simulink model "D53_LKAS_JLU_20200909_1612"  (R2018b)
settings: Solver=ode3  StartTime=0.0  StopTime=10.0  FixedStep=0.01  RelTol=1e-3  EnableMultiTasking=on
model workspace (MAT data in the model file):
  MCOS : class17 (value not decoded)
  MCOS : class17 (value not decoded)
  MCOS : class17 (value not decoded)
  MCOS : class17 (value not decoded)
  MCOS : class17 (value not decoded)
  MCOS : class17 (value not decoded)
  MCOS : class17 (value not decoded)
  MCOS : class17 (value not decoded)
  MCOS : class17 (value not decoded)
  MCOS : class17 (value not decoded)
  MCOS : class17 (value not decoded)
  MCOS : class17 (value not decoded)
  MCOS : class17 (value not decoded)
  MCOS : class17 (value not decoded)
  MCOS : class17 (value not decoded)
  MCOS : class17 (value not decoded)
  MCOS : class17 (value not decoded)
  MCOS : class17 (value not decoded)
  MCOS : class17 (value not decoded)
  MCOS : class17 (value not decoded)
  MCOS : class17 (value not decoded)
  MCOS : class17 (value not decoded)
  MCOS : class17 (value not decoded)
  MCOS : class17 (value not decoded)
  MCOS : class17 (value not decoded)
  MCOS : class17 (value not decoded)
  MCOS : class17 (value not decoded)
  MCOS : class17 (value not decoded)
  MCOS : class17 (value not decoded)
  MCOS : class17 (value not decoded)
  MCOS : class17 (value not decoded)
  MCOS : class17 (value not decoded)
  MCOS : class17 (value not decoded)
  MCOS : class17 (value not decoded)
  MCOS : class17 (value not decoded)
  MCOS : class17 (value not decoded)
  MCOS : class17 (value not decoded)
  MCOS : class17 (value not decoded)
  MCOS : class17 (value not decoded)
  MCOS : class17 (value not decoded)
  MCOS : class17 (value not decoded)
  MCOS : class17 (value not decoded)
  MCOS : class17 (value not decoded)
  MCOS : class17 (value not decoded)
  MCOS : class17 (value not decoded)
  MCOS : class17 (value not decoded)
  MCOS : class17 (value not decoded)
  MCOS : class17 (value not decoded)
  MCOS : class17 (value not decoded)
  MCOS : class17 (value not decoded)
  MCOS : class17 (value not decoded)
  MCOS : class17 (value not decoded)
  MCOS : class17 (value not decoded)
  MCOS : class17 (value not decoded)
  MCOS : class17 (value not decoded)
  MCOS : class17 (value not decoded)
  MCOS : class17 (value not decoded)
  MCOS : class17 (value not decoded)
  MCOS : class17 (value not decoded)
  MCOS : class17 (value not decoded)
  MCOS : class17 (value not decoded)
  MCOS : class17 (value not decoded)
  MCOS : class17 (value not decoded)
  MCOS : class17 (value not decoded)
  MCOS : class17 (value not decoded)
  MCOS : class17 (value not decoded)
  MCOS : class17 (value not decoded)
  MCOS : class17 (value not decoded)
  MCOS : class17 (value not decoded)
  MCOS : class17 (value not decoded)
  MCOS : class17 (value not decoded)
  MCOS : class17 (value not decoded)
  MCOS : class17 (value not decoded)
  MCOS : class17 (value not decoded)
  MCOS : class17 (value not decoded)
  MCOS : class17 (value not decoded)
  MCOS : class17 (value not decoded)
  MCOS : class17 (value not decoded)
  MCOS : class17 (value not decoded)
  MCOS : class17 (value not decoded)
  MCOS : class17 (value not decoded)
  MCOS : class17 (value not decoded)
  MCOS : class17 (value not decoded)
  MCOS : class17 (value not decoded)
  MCOS : class17 (value not decoded)
  MCOS : class17 (value not decoded)
  MCOS : class17 (value not decoded)
  MCOS : class17 (value not decoded)
  MCOS : class17 (value not decoded)
undefined symbols (not defined in the file): LKA_CarWidth, LKA_SampleTime, LKA_StrRatio_C, LKA_Veh2CamL_C, LKA_Veh2CamW_C, LKA_WhlBaseL_C, LL_CompSWA_C, LL_CrvtPrvwT_C, LL_DesDvt_C, LL_DvtComp_C, LL_DvtPrvwT_C, LL_DvtSpdDet_vDvtSpdMin_C, LL_HdAgExT_C, LL_HdAgPrvwT_C, LL_LAccMax_C, LL_LAccRMax_C, LL_LDW_EarliestWarnLine_C, LL_LDW_LatestWarnLine_C, LL_LDWS_SUPPRESS_HEADING, LL_LFClb_TFC_DiffCtlBalance, LL_LFClb_TFC_DiffCtrlMaxSWA, LL_LFClb_TFC_DiffCtrlRatio, LL_LFClb_TFC_facmGainLutGain1_C, LL_LFClb_TFC_facmGainLutGain2_C, LL_LFClb_TFC_facmIntegRatio, LL_LFClb_TFC_facmKlat_C, LL_LFClb_TFC_FfCtlRatio_C, LL_LFClb_TFC_phiIntegCtlMaxSWA_C, LL_LFClb_TFC_tiKlatPrvwT_C, LL_LFClb_TFC_vGainLutVehSpdLwr_C, LL_LFClb_TFC_vGainLutVehSpdUpr_C, LL_LKA_EarliestWarnLine_C, LL_LKA_LatestWarnLine_C, LL_LKAExPrcs_ExitC0Dvt, LL_LKAExPrcs_ExitC0Swt, LL_LKAExPrcs_tiExitTime1, LL_LKAExPrcs_tiExitTime2, LL_LKAExPrcs_tiExitTime3, LL_LKAS_OUT_OF_CONTROL_LAT_VEL, LL_LKAS_OUT_OF_CONTROL_TTLC, LL_LKASWASyn_M0, LL_LKASWASyn_M1, LL_LKASWASyn_M2, LL_LKASWASyn_M3K, LL_LKASWASyn_SWAaddMax, LL_LKASWASyn_T2, LL_LKASWASyn_tiTrqSwaRtTime, LL_LKASWASyn_tiTrqSwaTime, LL_LKASWASyn_TrqMax, LL_LKASWASyn_TrqSwaAddSwt, LL_LKASWASyn_TrqSwaRateDiff, LL_LSpdCompT_C, LL_lStpLngth_C, LL_MAX_DELAY_EPSSTAR_TIME, LL_MAX_DRIVER_TORQUE_DISABLE, LL_MAX_DRIVER_TORQUE_ENABLE, LL_MAX_LANE_WIDTH_DISABLE, LL_MAX_LANE_WIDTH_ENABLE, LL_MAX_LAT_ACC_DISABLE, LL_MAX_LAT_ACC_ENABLE ... (+30)
libraries: simulink x134, canmsglib x50, dspstat3 x3, simulink_extras x1
(part 2 of 17)

== system D53_LKAS_JLU_20200909_1612/CAN Monitor (CANMon)/Input ==
  In1 : Inport
  In2 : Inport  Port=2
  Bus Selector11 : BusSelector  OutputSignals=bsEPSInfo.EPS_LKA_State,bsEPSInfo.EPS_SW_Trq,bsSWAInfo.SW_Angle,bsSWAInfo.SW_Angle_Speed
  Bus Selector12 : BusSelector  OutputSignals=bsMP5Info.LKA_Main_Switch,bsMP5Info.LKA_Mode,bsPTState.TCU_ActualGear,bsLaneInfo.bsOriL0Info.O_L0_Q,bsLaneInfo.bsOriR0Info.O_R0_Q
  Bus Selector2 : BusSelector  OutputSignals=bsLaneInfo.bsOriL0Info.O_L0_C0,bsLaneInfo.bsOriL0Info.O_L0_C1,bsLaneInfo.bsOriL0Info.O_L0_C2,bsLaneInfo.bsOriL0Info.O_L0_TLC
  Bus Selector7 : BusSelector  OutputSignals=bsLaneInfo.bsOriR0Info.O_R0_C0,bsLaneInfo.bsOriR0Info.O_R0_C1,bsLaneInfo.bsOriR0Info.O_R0_C2,bsLaneInfo.bsOriR0Info.O_R0_TLC
  Bus Selector8 : BusSelector  OutputSignals=bsVehMovInfo.ESC_LatAcc,bsVehMovInfo.ESC_LonAcc,bsVehMovInfo.ESC_VehSpd,bsVehMovInfo.ESC_YawRate
  CAN Pack{16..19} (4 alike) : canmsglib/CAN Pack  CANdbFile=C:\Users\Administrator\Desktop\data_collect.dbc  MsgList=(none)  MsgName=c1deg  MsgIDType=Standard (11-bit identifier)  MsgIdentifier=2022  MsgLength=8  SignalInfo=EPSRx_trgSWTrq$8$16$2$2$1$0$0.01$0$-320$320$#EPSRx_stEPSCtlState$24$16$2$1$1$0$0.01$0$-320$320$#L0Range$40$16$2$1$1$0$1.000000e-002$0$-320$320$#R0Range$56$16$2$1$1$0$1.000000e-002$0$-320$320$#  NSignals=4  StartBits=str2num('[int32(8);int32(24);int32(40);int32(56)]')  SignalSizes=str2num('[int32(16);int32(16);int32(16);int32(16)]')  ByteOrders=str2num('[int32(2);int32(2);int32(2);int32(2)]')  DataTypes=str2num('[int32(2);int32(1);int32(1);int32(1)]')  MultiplexTypes=str2num('[int32(1);int32(1);int32(1);int32(1)]')  MultiplexValues=str2num('[double(0);double(0);double(0);double(0)]')  Factors=str2num('[double(0.01);double(0.01);double(1.000000e-002);double(1.000000e-002)]')  Offsets=str2num('[double(0);double(0);double(0);double(0)]')  Minimums=str2num('[double(-320);double(-320);double(-320);double(-320)]')  Maximums=str2num('[double(320);double(320);double(320);double(320)]')  Remote=off  ApplyMinMax=off  BusOutput=off
      settings: SourceProductName=Simulink Real-Time  SourceProductBaseCode=XP  DataFormat=manually specified signals
  CAN Pack20 : canmsglib/CAN Pack  CANdbFile=F:\LD\1_simulink\GateWay_20180716\dbc\camera_data_in.dbc  MsgList=(none)  MsgName=Video_Lane_Left_A  MsgIDType=Standard (11-bit identifier)  MsgIdentifier=1530  MsgLength=8  SignalInfo=C0$44$12$2$1$1$0$0.000001$0$-3$3$#C1$50$10$2$1$1$0$0.000001$0$-1$1$#C2$24$16$2$1$1$0$0.000001$0$-1$1$#C3$8$16$2$1$1$0$0.000001$0$-1$1$#Line_Type$59$3$2$2$1$0$1$0$0$7$#Message_Counter$48$2$2$2$1$0$1$0$0$3$#Quality$62$2$2$2$1$0$1$0$0$3$#  NSignals=7  StartBits=str2num('[int32(44);int32(50);int32(24);int32(8);int32(59);int32(48);int32(62)]')  SignalSizes=str2num('[int32(12);int32(10);int32(16);int32(16);int32(3);int32(2);int32(2)]')  ByteOrders=str2num('[int32(2);int32(2);int32(2);int32(2);int32(2);int32(2);int32(2)]')  DataTypes=str2num('[int32(1);int32(1);int32(1);int32(1);int32(2);int32(2);int32(2)]')  MultiplexTypes=str2num('[int32(1);int32(1);int32(1);int32(1);int32(1);int32(1);int32(1)]')  MultiplexValues=str2num('[double(0);double(0);double(0);double(0);double(0);double(0);double(0)]')  Factors=str2num('[double(0.000001);double(0.000001);double(0.000001);double(0.000001);double(1);double(1);double(1)]')  Offsets=str2num('[double(0);double(0);double(0);double(0);double(0);double(0);double(0)]')  Minimums=str2num('[double(-3);double(-1);double(-1);double(-1);double(0);double(0);double(0)]')  Maximums=str2num('[double(3);double(1);double(1);double(1);double(7);double(3);double(3)]')  Remote=off  ApplyMinMax=off  BusOutput=off
      settings: SourceProductName=Simulink Real-Time  SourceProductBaseCode=XP  DataFormat=manually specified signals
  CAN Send16 : S-Function  FunctionName=CAN_Send_P  Parameters=uint8(CAN_Port-1),uint8(CAN_Priority-1),uint8(S_overflow_flag),uint8(S_timestamp),double(sampletime)  SFunctionDeploymentMode=off  EnableBusSupport=off  mask{CAN_Port=CAN_0, CAN_Priority=3, S_overflow_flag=off, S_timestamp=off, sampletime=0.01}
      mask prompts: CAN_Port "CAN Port:"; CAN_Priority "Priority:"; S_overflow_flag "Send overflow flag"; S_timestamp "Send time stamp"
      mask init:
      | maskdisplay = cansendicon(CAN_Port,CAN_Priority,S_overflow_flag,S_timestamp);
      | set_param(gcb, 'MaskDisplay', maskdisplay);
      mask TypeOptions CAN_Port: CAN_0 | CAN_1 | CAN_2 | CAN_3
      mask TypeOptions CAN_Priority: 0 | 1 | 2 | 3 | 4 | 5 | 6 | 7
      mask Display: color('blue');text(0.98,0.9,'MPC5675K','horizontalAlignment','right');color('black');text(0.5,0.6,'FlexCAN_0 Send','horizontalAlignment','center');text(0.5,0.35,'Priority:3','horizontalAlignment','center');port_label('input',1,'CAN_Msg');
  CAN Send17 : S-Function  FunctionName=CAN_Send_P  Parameters=uint8(CAN_Port-1),uint8(CAN_Priority-1),uint8(S_overflow_flag),uint8(S_timestamp),double(sampletime)  SFunctionDeploymentMode=off  EnableBusSupport=off  mask{CAN_Port=CAN_0, CAN_Priority=3, S_overflow_flag=off, S_timestamp=off, sampletime=0.01}
      mask prompts: CAN_Port "CAN Port:"; CAN_Priority "Priority:"; S_overflow_flag "Send overflow flag"; S_timestamp "Send time stamp"
      mask init:
      | maskdisplay = cansendicon(CAN_Port,CAN_Priority,S_overflow_flag,S_timestamp);
      | set_param(gcb, 'MaskDisplay', maskdisplay);
      mask TypeOptions CAN_Port: CAN_0 | CAN_1 | CAN_2 | CAN_3
      mask TypeOptions CAN_Priority: 0 | 1 | 2 | 3 | 4 | 5 | 6 | 7
      mask Display: color('blue');text(0.98,0.9,'MPC5675K','horizontalAlignment','right');color('black');text(0.5,0.6,'FlexCAN_0 Send','horizontalAlignment','center');text(0.5,0.35,'Priority:3','horizontalAlignment','center');port_label('input',1,'CAN_Msg');
  CAN Send18 : S-Function  FunctionName=CAN_Send_P  Parameters=uint8(CAN_Port-1),uint8(CAN_Priority-1),uint8(S_overflow_flag),uint8(S_timestamp),double(sampletime)  SFunctionDeploymentMode=off  EnableBusSupport=off  mask{CAN_Port=CAN_0, CAN_Priority=3, S_overflow_flag=off, S_timestamp=off, sampletime=0.01}
      mask prompts: CAN_Port "CAN Port:"; CAN_Priority "Priority:"; S_overflow_flag "Send overflow flag"; S_timestamp "Send time stamp"
      mask init:
      | maskdisplay = cansendicon(CAN_Port,CAN_Priority,S_overflow_flag,S_timestamp);
      | set_param(gcb, 'MaskDisplay', maskdisplay);
      mask TypeOptions CAN_Port: CAN_0 | CAN_1 | CAN_2 | CAN_3
      mask TypeOptions CAN_Priority: 0 | 1 | 2 | 3 | 4 | 5 | 6 | 7
      mask Display: color('blue');text(0.98,0.9,'MPC5675K','horizontalAlignment','right');color('black');text(0.5,0.6,'FlexCAN_0 Send','horizontalAlignment','center');text(0.5,0.35,'Priority:3','horizontalAlignment','center');port_label('input',1,'CAN_Msg');
  CAN Send19 : S-Function  FunctionName=CAN_Send_P  Parameters=uint8(CAN_Port-1),uint8(CAN_Priority-1),uint8(S_overflow_flag),uint8(S_timestamp),double(sampletime)  SFunctionDeploymentMode=off  EnableBusSupport=off  mask{CAN_Port=CAN_0, CAN_Priority=3, S_overflow_flag=off, S_timestamp=off, sampletime=0.01}
      mask prompts: CAN_Port "CAN Port:"; CAN_Priority "Priority:"; S_overflow_flag "Send overflow flag"; S_timestamp "Send time stamp"
      mask init:
      | maskdisplay = cansendicon(CAN_Port,CAN_Priority,S_overflow_flag,S_timestamp);
      | set_param(gcb, 'MaskDisplay', maskdisplay);
      mask TypeOptions CAN_Port: CAN_0 | CAN_1 | CAN_2 | CAN_3
      mask TypeOptions CAN_Priority: 0 | 1 | 2 | 3 | 4 | 5 | 6 | 7
      mask Display: color('blue');text(0.98,0.9,'MPC5675K','horizontalAlignment','right');color('black');text(0.5,0.6,'FlexCAN_0 Send','horizontalAlignment','center');text(0.5,0.35,'Priority:3','horizontalAlignment','center');port_label('input',1,'CAN_Msg');
  CAN Send20 : S-Function  FunctionName=CAN_Send_P  Parameters=uint8(CAN_Port-1),uint8(CAN_Priority-1),uint8(S_overflow_flag),uint8(S_timestamp),double(sampletime)  SFunctionDeploymentMode=off  EnableBusSupport=off  mask{CAN_Port=CAN_0, CAN_Priority=3, S_overflow_flag=off, S_timestamp=off, sampletime=0.01}
      mask prompts: CAN_Port "CAN Port:"; CAN_Priority "Priority:"; S_overflow_flag "Send overflow flag"; S_timestamp "Send time stamp"
      mask init:
      | maskdisplay = cansendicon(CAN_Port,CAN_Priority,S_overflow_flag,S_timestamp);
      | set_param(gcb, 'MaskDisplay', maskdisplay);
      mask TypeOptions CAN_Port: CAN_0 | CAN_1 | CAN_2 | CAN_3
      mask TypeOptions CAN_Priority: 0 | 1 | 2 | 3 | 4 | 5 | 6 | 7
      mask Display: color('blue');text(0.98,0.9,'MPC5675K','horizontalAlignment','right');color('black');text(0.5,0.6,'FlexCAN_0 Send','horizontalAlignment','center');text(0.5,0.35,'Priority:3','horizontalAlignment','center');port_label('input',1,'CAN_Msg');
  Data Type Conversion{54..69} (16 alike) : DataTypeConversion  OutDataTypeStr=single
  Data Type Conversion{70..74} (5 alike) : DataTypeConversion  OutDataTypeStr=uint8
  wires:
  Data Type Conversion59/1 -> CAN Pack17/2
  Data Type Conversion60/1 -> CAN Pack17/3
  Bus Selector2/1 -> Data Type Conversion54/1  "<O_L0_C0>"
  Bus Selector12/1 -> Data Type Conversion70/1  "<LKA_Main_Switch>"
  CAN Pack18/1 -> CAN Send18/1
  Data Type Conversion66/1 -> CAN Pack19/1
  Data Type Conversion71/1 -> CAN Pack20/2
  [bsInInfo] -> Bus Selector7/1
  Data Type Conversion72/1 -> CAN Pack20/3
  Bus Selector12/4 -> Data Type Conversion73/1  "<O_L0_Q>"
  [bsInInfo] -> Bus Selector8/1
  Bus Selector2/2 -> Data Type Conversion55/1  "<O_L0_C1>"
  Data Type Conversion55/1 -> CAN Pack16/2
  Data Type Conversion57/1 -> CAN Pack16/4
  Bus Selector11/2 -> Data Type Conversion67/1  "<EPS_SW_Trq>"
  Bus Selector12/2 -> Data Type Conversion71/1  "<LKA_Mode>"
  Data Type Conversion61/1 -> CAN Pack17/4
  Bus Selector12/3 -> Data Type Conversion72/1  "<TCU_ActualGear>"
  In1/1 -> CAN Pack20/6
  Data Type Conversion64/1 -> CAN Pack18/3
  CAN Pack20/1 -> CAN Send20/1
  Bus Selector8/3 -> Data Type Conversion64/1  "<ESC_VehSpd>"
  Bus Selector8/4 -> Data Type Conversion65/1  "<ESC_YawRate>"
  Bus Selector7/1 -> Data Type Conversion58/1  "<O_R0_C0>"
  Bus Selector8/2 -> Data Type Conversion63/1  "<ESC_LonAcc>"
  In2/1 -> CAN Pack20/7
  Bus Selector7/2 -> Data Type Conversion59/1  "<O_R0_C1>"
  Bus Selector7/4 -> Data Type Conversion61/1  "<O_R0_TLC>"
  Bus Selector11/3 -> Data Type Conversion68/1  "<SW_Angle>"
  Bus Selector11/4 -> Data Type Conversion69/1  "<SW_Angle_Speed>"
  CAN Pack16/1 -> CAN Send16/1
  Data Type Conversion56/1 -> CAN Pack16/3
  Data Type Conversion70/1 -> CAN Pack20/1
  Bus Selector11/1 -> Data Type Conversion66/1  "<EPS_LKA_State>"
  Bus Selector2/3 -> Data Type Conversion56/1  "<O_L0_C2>"
  Bus Selector12/5 -> Data Type Conversion74/1  "<O_R0_Q>"
  Bus Selector8/1 -> Data Type Conversion62/1  "<ESC_LatAcc>"
  CAN Pack17/1 -> CAN Send17/1
  [bsInInfo] -> Bus Selector11/1
  Data Type Conversion58/1 -> CAN Pack17/1
  [bsInInfo] -> Bus Selector2/1
  Bus Selector7/3 -> Data Type Conversion60/1  "<O_R0_C2>"
  Bus Selector2/4 -> Data Type Conversion57/1  "<O_L0_TLC>"
  Data Type Conversion68/1 -> CAN Pack19/3
  Data Type Conversion54/1 -> CAN Pack16/1
  Data Type Conversion74/1 -> CAN Pack20/5
  CAN Pack19/1 -> CAN Send19/1
  [bsInInfo] -> Bus Selector12/1
  Data Type Conversion65/1 -> CAN Pack18/4
  Data Type Conversion63/1 -> CAN Pack18/2
  Data Type Conversion73/1 -> CAN Pack20/4
  Data Type Conversion67/1 -> CAN Pack19/2
  Data Type Conversion69/1 -> CAN Pack19/4
  Data Type Conversion62/1 -> CAN Pack18/1

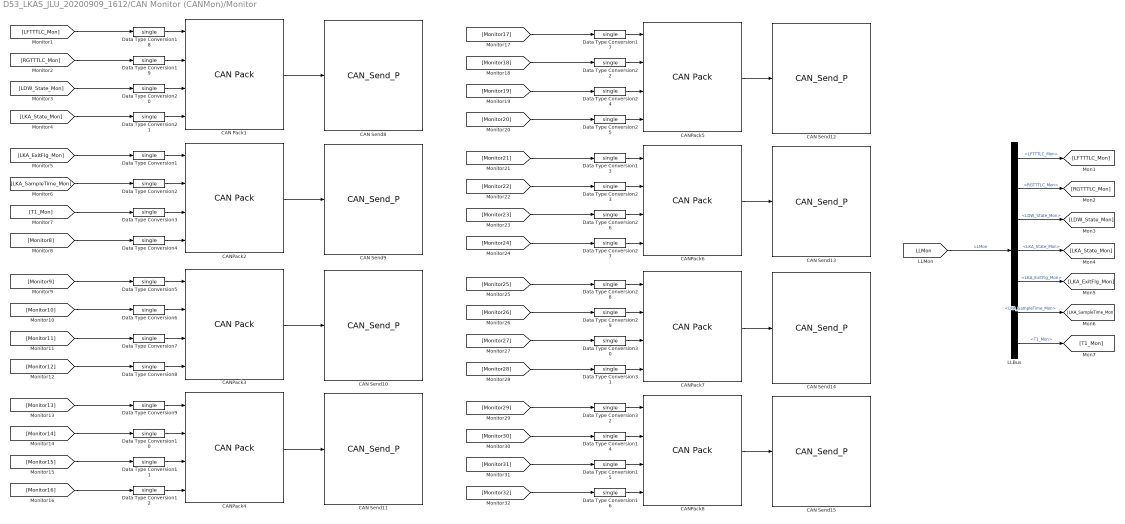
== system D53_LKAS_JLU_20200909_1612/CAN Monitor (CANMon)/Monitor ==
  CAN Pack1 : canmsglib/CAN Pack  CANdbFile=D:\LKAS\Documents\LKAS-Monitor.dbc  MsgList=Mon_1  MsgName=Mon_1  MsgIDType=Standard (11-bit identifier)  MsgIdentifier=1536  MsgLength=8  SignalInfo=Signal_1$8$16$2$1$1$0$1.000000e-02$0$-3.276800e+02$3.276700e+02$#Signal_2$24$16$2$1$1$0$1.000000e-02$0$-3.276800e+02$3.276700e+02$#Signal_3$40$16$2$1$1$0$1.000000e-02$0$-3.276800e+02$3.276700e+02$#Signal_4$56$16$2$1$1$0$1.000000e-02$0$-3.276800e+02$3.276700e+02$#  NSignals=4  StartBits=str2num('[int32(8);int32(24);int32(40);int32(56)]')  SignalSizes=str2num('[int32(16);int32(16);int32(16);int32(16)]')  ByteOrders=str2num('[int32(2);int32(2);int32(2);int32(2)]')  DataTypes=str2num('[int32(1);int32(1);int32(1);int32(1)]')  MultiplexTypes=str2num('[int32(1);int32(1);int32(1);int32(1)]')  MultiplexValues=str2num('[double(0);double(0);double(0);double(0)]')  Factors=str2num('[double(1.000000e-02);double(1.000000e-02);double(1.000000e-02);double(1.000000e-02)]')  Offsets=str2num('[double(0);double(0);double(0);double(0)]')  Minimums=str2num('[double(-3.276800e+02);double(-3.276800e+02);double(-3.276800e+02);double(-3.276800e+02)]')  Maximums=str2num('[double(3.276700e+02);double(3.276700e+02);double(3.276700e+02);double(3.276700e+02)]')  Remote=off  ApplyMinMax=off  BusOutput=off
      settings: SourceProductName=Simulink Real-Time  SourceProductBaseCode=XP  DataFormat=CANdb specified signals
  CAN Send10 : S-Function  FunctionName=CAN_Send_P  Parameters=uint8(CAN_Port-1),uint8(CAN_Priority-1),uint8(S_overflow_flag),uint8(S_timestamp),double(sampletime)  SFunctionDeploymentMode=off  EnableBusSupport=off  mask{CAN_Port=CAN_0, CAN_Priority=3, S_overflow_flag=off, S_timestamp=off, sampletime=0.01}
      mask prompts: CAN_Port "CAN Port:"; CAN_Priority "Priority:"; S_overflow_flag "Send overflow flag"; S_timestamp "Send time stamp"
      mask init:
      | maskdisplay = cansendicon(CAN_Port,CAN_Priority,S_overflow_flag,S_timestamp);
      | set_param(gcb, 'MaskDisplay', maskdisplay);
      mask TypeOptions CAN_Port: CAN_0 | CAN_1 | CAN_2 | CAN_3
      mask TypeOptions CAN_Priority: 0 | 1 | 2 | 3 | 4 | 5 | 6 | 7
      mask Display: color('blue');text(0.98,0.9,'MPC5675K','horizontalAlignment','right');color('black');text(0.5,0.6,'FlexCAN_0 Send','horizontalAlignment','center');text(0.5,0.35,'Priority:3','horizontalAlignment','center');port_label('input',1,'CAN_Msg');
  CAN Send11 : S-Function  FunctionName=CAN_Send_P  Parameters=uint8(CAN_Port-1),uint8(CAN_Priority-1),uint8(S_overflow_flag),uint8(S_timestamp),double(sampletime)  SFunctionDeploymentMode=off  EnableBusSupport=off  mask{CAN_Port=CAN_0, CAN_Priority=3, S_overflow_flag=off, S_timestamp=off, sampletime=0.01}
      mask prompts: CAN_Port "CAN Port:"; CAN_Priority "Priority:"; S_overflow_flag "Send overflow flag"; S_timestamp "Send time stamp"
      mask init:
      | maskdisplay = cansendicon(CAN_Port,CAN_Priority,S_overflow_flag,S_timestamp);
      | set_param(gcb, 'MaskDisplay', maskdisplay);
      mask TypeOptions CAN_Port: CAN_0 | CAN_1 | CAN_2 | CAN_3
      mask TypeOptions CAN_Priority: 0 | 1 | 2 | 3 | 4 | 5 | 6 | 7
      mask Display: color('blue');text(0.98,0.9,'MPC5675K','horizontalAlignment','right');color('black');text(0.5,0.6,'FlexCAN_0 Send','horizontalAlignment','center');text(0.5,0.35,'Priority:3','horizontalAlignment','center');port_label('input',1,'CAN_Msg');
  CAN Send12 : S-Function  FunctionName=CAN_Send_P  Parameters=uint8(CAN_Port-1),uint8(CAN_Priority-1),uint8(S_overflow_flag),uint8(S_timestamp),double(sampletime)  SFunctionDeploymentMode=off  EnableBusSupport=off  mask{CAN_Port=CAN_0, CAN_Priority=3, S_overflow_flag=off, S_timestamp=off, sampletime=0.01}
      mask prompts: CAN_Port "CAN Port:"; CAN_Priority "Priority:"; S_overflow_flag "Send overflow flag"; S_timestamp "Send time stamp"
      mask init:
      | maskdisplay = cansendicon(CAN_Port,CAN_Priority,S_overflow_flag,S_timestamp);
      | set_param(gcb, 'MaskDisplay', maskdisplay);
      mask TypeOptions CAN_Port: CAN_0 | CAN_1 | CAN_2 | CAN_3
      mask TypeOptions CAN_Priority: 0 | 1 | 2 | 3 | 4 | 5 | 6 | 7
      mask Display: color('blue');text(0.98,0.9,'MPC5675K','horizontalAlignment','right');color('black');text(0.5,0.6,'FlexCAN_0 Send','horizontalAlignment','center');text(0.5,0.35,'Priority:3','horizontalAlignment','center');port_label('input',1,'CAN_Msg');
  CAN Send13 : S-Function  FunctionName=CAN_Send_P  Parameters=uint8(CAN_Port-1),uint8(CAN_Priority-1),uint8(S_overflow_flag),uint8(S_timestamp),double(sampletime)  SFunctionDeploymentMode=off  EnableBusSupport=off  mask{CAN_Port=CAN_0, CAN_Priority=3, S_overflow_flag=off, S_timestamp=off, sampletime=0.01}
      mask prompts: CAN_Port "CAN Port:"; CAN_Priority "Priority:"; S_overflow_flag "Send overflow flag"; S_timestamp "Send time stamp"
      mask init:
      | maskdisplay = cansendicon(CAN_Port,CAN_Priority,S_overflow_flag,S_timestamp);
      | set_param(gcb, 'MaskDisplay', maskdisplay);
      mask TypeOptions CAN_Port: CAN_0 | CAN_1 | CAN_2 | CAN_3
      mask TypeOptions CAN_Priority: 0 | 1 | 2 | 3 | 4 | 5 | 6 | 7
      mask Display: color('blue');text(0.98,0.9,'MPC5675K','horizontalAlignment','right');color('black');text(0.5,0.6,'FlexCAN_0 Send','horizontalAlignment','center');text(0.5,0.35,'Priority:3','horizontalAlignment','center');port_label('input',1,'CAN_Msg');
  CAN Send14 : S-Function  FunctionName=CAN_Send_P  Parameters=uint8(CAN_Port-1),uint8(CAN_Priority-1),uint8(S_overflow_flag),uint8(S_timestamp),double(sampletime)  SFunctionDeploymentMode=off  EnableBusSupport=off  mask{CAN_Port=CAN_0, CAN_Priority=3, S_overflow_flag=off, S_timestamp=off, sampletime=0.01}
      mask prompts: CAN_Port "CAN Port:"; CAN_Priority "Priority:"; S_overflow_flag "Send overflow flag"; S_timestamp "Send time stamp"
      mask init:
      | maskdisplay = cansendicon(CAN_Port,CAN_Priority,S_overflow_flag,S_timestamp);
      | set_param(gcb, 'MaskDisplay', maskdisplay);
      mask TypeOptions CAN_Port: CAN_0 | CAN_1 | CAN_2 | CAN_3
      mask TypeOptions CAN_Priority: 0 | 1 | 2 | 3 | 4 | 5 | 6 | 7
      mask Display: color('blue');text(0.98,0.9,'MPC5675K','horizontalAlignment','right');color('black');text(0.5,0.6,'FlexCAN_0 Send','horizontalAlignment','center');text(0.5,0.35,'Priority:3','horizontalAlignment','center');port_label('input',1,'CAN_Msg');
  CAN Send15 : S-Function  FunctionName=CAN_Send_P  Parameters=uint8(CAN_Port-1),uint8(CAN_Priority-1),uint8(S_overflow_flag),uint8(S_timestamp),double(sampletime)  SFunctionDeploymentMode=off  EnableBusSupport=off  mask{CAN_Port=CAN_0, CAN_Priority=3, S_overflow_flag=off, S_timestamp=off, sampletime=0.01}
      mask prompts: CAN_Port "CAN Port:"; CAN_Priority "Priority:"; S_overflow_flag "Send overflow flag"; S_timestamp "Send time stamp"
      mask init:
      | maskdisplay = cansendicon(CAN_Port,CAN_Priority,S_overflow_flag,S_timestamp);
      | set_param(gcb, 'MaskDisplay', maskdisplay);
      mask TypeOptions CAN_Port: CAN_0 | CAN_1 | CAN_2 | CAN_3
      mask TypeOptions CAN_Priority: 0 | 1 | 2 | 3 | 4 | 5 | 6 | 7
      mask Display: color('blue');text(0.98,0.9,'MPC5675K','horizontalAlignment','right');color('black');text(0.5,0.6,'FlexCAN_0 Send','horizontalAlignment','center');text(0.5,0.35,'Priority:3','horizontalAlignment','center');port_label('input',1,'CAN_Msg');
  CAN Send8 : S-Function  FunctionName=CAN_Send_P  Parameters=uint8(CAN_Port-1),uint8(CAN_Priority-1),uint8(S_overflow_flag),uint8(S_timestamp),double(sampletime)  SFunctionDeploymentMode=off  EnableBusSupport=off  mask{CAN_Port=CAN_0, CAN_Priority=3, S_overflow_flag=off, S_timestamp=off, sampletime=0.01}
      mask prompts: CAN_Port "CAN Port:"; CAN_Priority "Priority:"; S_overflow_flag "Send overflow flag"; S_timestamp "Send time stamp"
      mask init:
      | maskdisplay = cansendicon(CAN_Port,CAN_Priority,S_overflow_flag,S_timestamp);
      | set_param(gcb, 'MaskDisplay', maskdisplay);
      mask TypeOptions CAN_Port: CAN_0 | CAN_1 | CAN_2 | CAN_3
      mask TypeOptions CAN_Priority: 0 | 1 | 2 | 3 | 4 | 5 | 6 | 7
      mask Display: color('blue');text(0.98,0.9,'MPC5675K','horizontalAlignment','right');color('black');text(0.5,0.6,'FlexCAN_0 Send','horizontalAlignment','center');text(0.5,0.35,'Priority:3','horizontalAlignment','center');port_label('input',1,'CAN_Msg');
  CAN Send9 : S-Function  FunctionName=CAN_Send_P  Parameters=uint8(CAN_Port-1),uint8(CAN_Priority-1),uint8(S_overflow_flag),uint8(S_timestamp),double(sampletime)  SFunctionDeploymentMode=off  EnableBusSupport=off  mask{CAN_Port=CAN_0, CAN_Priority=3, S_overflow_flag=off, S_timestamp=off, sampletime=0.01}
      mask prompts: CAN_Port "CAN Port:"; CAN_Priority "Priority:"; S_overflow_flag "Send overflow flag"; S_timestamp "Send time stamp"
      mask init:
      | maskdisplay = cansendicon(CAN_Port,CAN_Priority,S_overflow_flag,S_timestamp);
      | set_param(gcb, 'MaskDisplay', maskdisplay);
      mask TypeOptions CAN_Port: CAN_0 | CAN_1 | CAN_2 | CAN_3
      mask TypeOptions CAN_Priority: 0 | 1 | 2 | 3 | 4 | 5 | 6 | 7
      mask Display: color('blue');text(0.98,0.9,'MPC5675K','horizontalAlignment','right');color('black');text(0.5,0.6,'FlexCAN_0 Send','horizontalAlignment','center');text(0.5,0.35,'Priority:3','horizontalAlignment','center');port_label('input',1,'CAN_Msg');
  CANPack2 : canmsglib/CAN Pack  CANdbFile=D:\LKAS\Documents\LKAS-Monitor.dbc  MsgList=Mon_2  MsgName=Mon_2  MsgIDType=Standard (11-bit identifier)  MsgIdentifier=1552  MsgLength=8  SignalInfo=bsInInfo1$8$16$2$1$1$0$1.000000e-02$0$-3.276800e+02$3.276700e+02$#bsInInfo2$24$16$2$1$1$0$1.000000e-02$0$-3.276800e+02$3.276700e+02$#bsInInfo3$40$16$2$1$1$0$1.000000e-02$0$-3.276800e+02$3.276700e+02$#bsInInfo4$56$16$2$1$1$0$1.000000e-02$0$-3.276800e+02$3.276700e+02$#  NSignals=4  StartBits=str2num('[int32(8);int32(24);int32(40);int32(56)]')  SignalSizes=str2num('[int32(16);int32(16);int32(16);int32(16)]')  ByteOrders=str2num('[int32(2);int32(2);int32(2);int32(2)]')  DataTypes=str2num('[int32(1);int32(1);int32(1);int32(1)]')  MultiplexTypes=str2num('[int32(1);int32(1);int32(1);int32(1)]')  MultiplexValues=str2num('[double(0);double(0);double(0);double(0)]')  Factors=str2num('[double(1.000000e-02);double(1.000000e-02);double(1.000000e-02);double(1.000000e-02)]')  Offsets=str2num('[double(0);double(0);double(0);double(0)]')  Minimums=str2num('[double(-3.276800e+02);double(-3.276800e+02);double(-3.276800e+02);double(-3.276800e+02)]')  Maximums=str2num('[double(3.276700e+02);double(3.276700e+02);double(3.276700e+02);double(3.276700e+02)]')  Remote=off  ApplyMinMax=off  BusOutput=off
      settings: SourceProductName=Simulink Real-Time  SourceProductBaseCode=XP  DataFormat=CANdb specified signals
  CANPack3 : canmsglib/CAN Pack  CANdbFile=D:\LKAS\Documents\LKAS-Monitor.dbc  MsgList=Mon_3  MsgName=Mon_3  MsgIDType=Standard (11-bit identifier)  MsgIdentifier=1568  MsgLength=8  SignalInfo=Signal_10$24$16$2$1$1$0$1.000000e-02$0$-3.276800e+02$3.276700e+02$#Signal_11$40$16$2$1$1$0$1.000000e-02$0$-3.276800e+02$3.276700e+02$#Signal_12$56$16$2$1$1$0$1.000000e-02$0$-3.276800e+02$3.276700e+02$#Signal_9$8$16$2$1$1$0$1.000000e-02$0$-3.276800e+02$3.276700e+02$#  NSignals=4  StartBits=str2num('[int32(24);int32(40);int32(56);int32(8)]')  SignalSizes=str2num('[int32(16);int32(16);int32(16);int32(16)]')  ByteOrders=str2num('[int32(2);int32(2);int32(2);int32(2)]')  DataTypes=str2num('[int32(1);int32(1);int32(1);int32(1)]')  MultiplexTypes=str2num('[int32(1);int32(1);int32(1);int32(1)]')  MultiplexValues=str2num('[double(0);double(0);double(0);double(0)]')  Factors=str2num('[double(1.000000e-02);double(1.000000e-02);double(1.000000e-02);double(1.000000e-02)]')  Offsets=str2num('[double(0);double(0);double(0);double(0)]')  Minimums=str2num('[double(-3.276800e+02);double(-3.276800e+02);double(-3.276800e+02);double(-3.276800e+02)]')  Maximums=str2num('[double(3.276700e+02);double(3.276700e+02);double(3.276700e+02);double(3.276700e+02)]')  Remote=off  ApplyMinMax=off  BusOutput=off
      settings: SourceProductName=Simulink Real-Time  SourceProductBaseCode=XP  DataFormat=CANdb specified signals
  CANPack4 : canmsglib/CAN Pack  CANdbFile=D:\LKAS\Documents\LKAS-Monitor.dbc  MsgList=Mon_4  MsgName=Mon_4  MsgIDType=Standard (11-bit identifier)  MsgIdentifier=1584  MsgLength=8  SignalInfo=Signal_13$8$16$2$1$1$0$1.000000e-02$0$-3.276800e+02$3.276700e+02$#Signal_14$24$16$2$1$1$0$1.000000e-02$0$-3.276800e+02$3.276700e+02$#Signal_15$40$16$2$1$1$0$1.000000e-02$0$-3.276800e+02$3.276700e+02$#Signal_16$56$16$2$1$1$0$1.000000e-02$0$-3.276800e+02$3.276700e+02$#  NSignals=4  StartBits=str2num('[int32(8);int32(24);int32(40);int32(56)]')  SignalSizes=str2num('[int32(16);int32(16);int32(16);int32(16)]')  ByteOrders=str2num('[int32(2);int32(2);int32(2);int32(2)]')  DataTypes=str2num('[int32(1);int32(1);int32(1);int32(1)]')  MultiplexTypes=str2num('[int32(1);int32(1);int32(1);int32(1)]')  MultiplexValues=str2num('[double(0);double(0);double(0);double(0)]')  Factors=str2num('[double(1.000000e-02);double(1.000000e-02);double(1.000000e-02);double(1.000000e-02)]')  Offsets=str2num('[double(0);double(0);double(0);double(0)]')  Minimums=str2num('[double(-3.276800e+02);double(-3.276800e+02);double(-3.276800e+02);double(-3.276800e+02)]')  Maximums=str2num('[double(3.276700e+02);double(3.276700e+02);double(3.276700e+02);double(3.276700e+02)]')  Remote=off  ApplyMinMax=off  BusOutput=off
      settings: SourceProductName=Simulink Real-Time  SourceProductBaseCode=XP  DataFormat=CANdb specified signals
  CANPack5 : canmsglib/CAN Pack  CANdbFile=D:\LKAS\Documents\LKAS-Monitor.dbc  MsgList=Mon_5  MsgName=Mon_5  MsgIDType=Standard (11-bit identifier)  MsgIdentifier=1600  MsgLength=8  SignalInfo=Signal_17$8$16$2$1$1$0$1.000000e-02$0$-3.276800e+02$3.276700e+02$#Signal_18$24$16$2$1$1$0$1.000000e-02$0$-3.276800e+02$3.276700e+02$#Signal_19$40$16$2$1$1$0$1.000000e-02$0$-3.276800e+02$3.276700e+02$#Signal_20$56$16$2$1$1$0$1.000000e-02$0$-3.276800e+02$3.276700e+02$#  NSignals=4  StartBits=str2num('[int32(8);int32(24);int32(40);int32(56)]')  SignalSizes=str2num('[int32(16);int32(16);int32(16);int32(16)]')  ByteOrders=str2num('[int32(2);int32(2);int32(2);int32(2)]')  DataTypes=str2num('[int32(1);int32(1);int32(1);int32(1)]')  MultiplexTypes=str2num('[int32(1);int32(1);int32(1);int32(1)]')  MultiplexValues=str2num('[double(0);double(0);double(0);double(0)]')  Factors=str2num('[double(1.000000e-02);double(1.000000e-02);double(1.000000e-02);double(1.000000e-02)]')  Offsets=str2num('[double(0);double(0);double(0);double(0)]')  Minimums=str2num('[double(-3.276800e+02);double(-3.276800e+02);double(-3.276800e+02);double(-3.276800e+02)]')  Maximums=str2num('[double(3.276700e+02);double(3.276700e+02);double(3.276700e+02);double(3.276700e+02)]')  Remote=off  ApplyMinMax=off  BusOutput=off
      settings: SourceProductName=Simulink Real-Time  SourceProductBaseCode=XP  DataFormat=CANdb specified signals
  CANPack6 : canmsglib/CAN Pack  CANdbFile=D:\LKAS\Documents\LKAS-Monitor.dbc  MsgList=Mon_6  MsgName=Mon_6  MsgIDType=Standard (11-bit identifier)  MsgIdentifier=1616  MsgLength=8  SignalInfo=Signal_21$8$16$2$1$1$0$1.000000e-02$0$-3.276800e+02$3.276700e+02$#Signal_22$24$16$2$1$1$0$1.000000e-02$0$-3.276800e+02$3.276700e+02$#Signal_23$40$16$2$1$1$0$1.000000e-02$0$-3.276800e+02$3.276700e+02$#Signal_24$56$16$2$1$1$0$1.000000e-02$0$-3.276800e+02$3.276700e+02$#  NSignals=4  StartBits=str2num('[int32(8);int32(24);int32(40);int32(56)]')  SignalSizes=str2num('[int32(16);int32(16);int32(16);int32(16)]')  ByteOrders=str2num('[int32(2);int32(2);int32(2);int32(2)]')  DataTypes=str2num('[int32(1);int32(1);int32(1);int32(1)]')  MultiplexTypes=str2num('[int32(1);int32(1);int32(1);int32(1)]')  MultiplexValues=str2num('[double(0);double(0);double(0);double(0)]')  Factors=str2num('[double(1.000000e-02);double(1.000000e-02);double(1.000000e-02);double(1.000000e-02)]')  Offsets=str2num('[double(0);double(0);double(0);double(0)]')  Minimums=str2num('[double(-3.276800e+02);double(-3.276800e+02);double(-3.276800e+02);double(-3.276800e+02)]')  Maximums=str2num('[double(3.276700e+02);double(3.276700e+02);double(3.276700e+02);double(3.276700e+02)]')  Remote=off  ApplyMinMax=off  BusOutput=off
      settings: SourceProductName=Simulink Real-Time  SourceProductBaseCode=XP  DataFormat=CANdb specified signals
  CANPack7 : canmsglib/CAN Pack  CANdbFile=D:\LKAS\Documents\LKAS-Monitor.dbc  MsgList=Mon_7  MsgName=Mon_7  MsgIDType=Standard (11-bit identifier)  MsgIdentifier=1632  MsgLength=8  SignalInfo=Signal_25$8$16$2$1$1$0$1.000000e-02$0$-3.276800e+02$3.276700e+02$#Signal_26$24$16$2$1$1$0$1.000000e-02$0$-3.276800e+02$3.276700e+02$#Signal_27$40$16$2$1$1$0$1.000000e-02$0$-3.276800e+02$3.276700e+02$#Signal_28$56$16$2$1$1$0$1.000000e-02$0$-3.276800e+02$3.276700e+02$#  NSignals=4  StartBits=str2num('[int32(8);int32(24);int32(40);int32(56)]')  SignalSizes=str2num('[int32(16);int32(16);int32(16);int32(16)]')  ByteOrders=str2num('[int32(2);int32(2);int32(2);int32(2)]')  DataTypes=str2num('[int32(1);int32(1);int32(1);int32(1)]')  MultiplexTypes=str2num('[int32(1);int32(1);int32(1);int32(1)]')  MultiplexValues=str2num('[double(0);double(0);double(0);double(0)]')  Factors=str2num('[double(1.000000e-02);double(1.000000e-02);double(1.000000e-02);double(1.000000e-02)]')  Offsets=str2num('[double(0);double(0);double(0);double(0)]')  Minimums=str2num('[double(-3.276800e+02);double(-3.276800e+02);double(-3.276800e+02);double(-3.276800e+02)]')  Maximums=str2num('[double(3.276700e+02);double(3.276700e+02);double(3.276700e+02);double(3.276700e+02)]')  Remote=off  ApplyMinMax=off  BusOutput=off
      settings: SourceProductName=Simulink Real-Time  SourceProductBaseCode=XP  DataFormat=CANdb specified signals
  CANPack8 : canmsglib/CAN Pack  CANdbFile=D:\LKAS\Documents\LKAS-Monitor.dbc  MsgList=Mon_8  MsgName=Mon_8  MsgIDType=Standard (11-bit identifier)  MsgIdentifier=1648  MsgLength=8  SignalInfo=Signal_29$8$16$2$1$1$0$1.000000e-02$0$-3.276800e+02$3.276700e+02$#Signal_30$24$16$2$1$1$0$1.000000e-02$0$-3.276800e+02$3.276700e+02$#Signal_31$40$16$2$1$1$0$1.000000e-02$0$-3.276800e+02$3.276700e+02$#Signal_32$56$16$2$1$1$0$1.000000e-02$0$-3.276800e+02$3.276700e+02$#  NSignals=4  StartBits=str2num('[int32(8);int32(24);int32(40);int32(56)]')  SignalSizes=str2num('[int32(16);int32(16);int32(16);int32(16)]')  ByteOrders=str2num('[int32(2);int32(2);int32(2);int32(2)]')  DataTypes=str2num('[int32(1);int32(1);int32(1);int32(1)]')  MultiplexTypes=str2num('[int32(1);int32(1);int32(1);int32(1)]')  MultiplexValues=str2num('[double(0);double(0);double(0);double(0)]')  Factors=str2num('[double(1.000000e-02);double(1.000000e-02);double(1.000000e-02);double(1.000000e-02)]')  Offsets=str2num('[double(0);double(0);double(0);double(0)]')  Minimums=str2num('[double(-3.276800e+02);double(-3.276800e+02);double(-3.276800e+02);double(-3.276800e+02)]')  Maximums=str2num('[double(3.276700e+02);double(3.276700e+02);double(3.276700e+02);double(3.276700e+02)]')  Remote=off  ApplyMinMax=off  BusOutput=off
      settings: SourceProductName=Simulink Real-Time  SourceProductBaseCode=XP  DataFormat=CANdb specified signals
  Data Type Conversion{1..32} (32 alike) : DataTypeConversion  OutDataTypeStr=single
  LLBus : BusSelector  OutputSignals=InPMon.LFTTTLC_Mon,InPMon.RGTTTLC_Mon,StateMon.LDW_State_Mon,StateMon.LKA_State_Mon,LKAMon.LKA_ExitFlg_Mon,LKAMon.LKA_SampleTime_Mon,LKAMon.T1_Mon
  wires:
  CANPack3/1 -> CAN Send10/1
  Data Type Conversion21/1 -> CAN Pack1/4
  [LDW_State_Mon] -> Data Type Conversion20/1
  CANPack5/1 -> CAN Send12/1
  CANPack7/1 -> CAN Send14/1
  CAN Pack1/1 -> CAN Send8/1
  Data Type Conversion18/1 -> CAN Pack1/1
  Data Type Conversion19/1 -> CAN Pack1/2
  CANPack6/1 -> CAN Send13/1
  [RGTTTLC_Mon] -> Data Type Conversion19/1
  [LKA_State_Mon] -> Data Type Conversion21/1
  CANPack4/1 -> CAN Send11/1
  CANPack8/1 -> CAN Send15/1
  CANPack2/1 -> CAN Send9/1
  Data Type Conversion20/1 -> CAN Pack1/3
  [LFTTTLC_Mon] -> Data Type Conversion18/1
  [LKA_ExitFlg_Mon] -> Data Type Conversion1/1
  Data Type Conversion3/1 -> CANPack2/3
  [Monitor8] -> Data Type Conversion4/1
  [LKA_SampleTime_Mon] -> Data Type Conversion2/1
  Data Type Conversion2/1 -> CANPack2/2
  Data Type Conversion1/1 -> CANPack2/1
  [T1_Mon] -> Data Type Conversion3/1
  Data Type Conversion4/1 -> CANPack2/4
  Data Type Conversion8/1 -> CANPack3/4
  [Monitor11] -> Data Type Conversion7/1
  Data Type Conversion5/1 -> CANPack3/1
  Data Type Conversion6/1 -> CANPack3/2
  [Monitor10] -> Data Type Conversion6/1
  [Monitor12] -> Data Type Conversion8/1
  Data Type Conversion7/1 -> CANPack3/3
  [Monitor9] -> Data Type Conversion5/1
  [Monitor13] -> Data Type Conversion9/1
  Data Type Conversion11/1 -> CANPack4/3
  [Monitor16] -> Data Type Conversion12/1
  [Monitor14] -> Data Type Conversion10/1
  Data Type Conversion10/1 -> CANPack4/2
  Data Type Conversion9/1 -> CANPack4/1
  [Monitor15] -> Data Type Conversion11/1
  Data Type Conversion12/1 -> CANPack4/4
  Data Type Conversion16/1 -> CANPack8/4
  [Monitor31] -> Data Type Conversion15/1
  Data Type Conversion32/1 -> CANPack8/1
  Data Type Conversion14/1 -> CANPack8/2
  [Monitor30] -> Data Type Conversion14/1
  [Monitor32] -> Data Type Conversion16/1
  Data Type Conversion15/1 -> CANPack8/3
  [Monitor29] -> Data Type Conversion32/1
  [Monitor25] -> Data Type Conversion28/1
  Data Type Conversion30/1 -> CANPack7/3
  [Monitor28] -> Data Type Conversion31/1
  [Monitor26] -> Data Type Conversion29/1
  Data Type Conversion29/1 -> CANPack7/2
  Data Type Conversion28/1 -> CANPack7/1
  [Monitor27] -> Data Type Conversion30/1
  Data Type Conversion31/1 -> CANPack7/4
  Data Type Conversion27/1 -> CANPack6/4
  [Monitor23] -> Data Type Conversion26/1
  Data Type Conversion13/1 -> CANPack6/1
  Data Type Conversion23/1 -> CANPack6/2
  [Monitor22] -> Data Type Conversion23/1
  [Monitor24] -> Data Type Conversion27/1
  Data Type Conversion26/1 -> CANPack6/3
  [Monitor21] -> Data Type Conversion13/1
  [Monitor17] -> Data Type Conversion17/1
  Data Type Conversion24/1 -> CANPack5/3
  [Monitor20] -> Data Type Conversion25/1
  [Monitor18] -> Data Type Conversion22/1
  Data Type Conversion22/1 -> CANPack5/2
  Data Type Conversion17/1 -> CANPack5/1
  [Monitor19] -> Data Type Conversion24/1
  Data Type Conversion25/1 -> CANPack5/4
  [LLMon] -> LLBus/1  "LLMon"
  LLBus/1 -> [LFTTTLC_Mon]  "<LFTTTLC_Mon>"
  LLBus/2 -> [RGTTTLC_Mon]  "<RGTTTLC_Mon>"
  LLBus/3 -> [LDW_State_Mon]  "<LDW_State_Mon>"
  LLBus/4 -> [LKA_State_Mon]  "<LKA_State_Mon>"
  LLBus/5 -> [LKA_ExitFlg_Mon]  "<LKA_ExitFlg_Mon>"
  LLBus/6 -> [LKA_SampleTime_Mon]  "<LKA_SampleTime_Mon>"
  LLBus/7 -> [T1_Mon]  "<T1_Mon>"

== system D53_LKAS_JLU_20200909_1612/CAN Monitor (CANMon)/Output ==
  Bus Selector13 : BusSelector  OutputSignals=LMS_phiSWACmd,EPS_State_Ctl,Coefficient_toregulate_EPS,Permit_to_know_if_LKA_or_LPA3F2,LDW_Flag,LDW_Status_Display,LKA_action_indication,LKA_Status_Display,HMI_Popup_Status,Hands_off_warning,Vehicle_Lane_Display
  CAN Pack21 : canmsglib/CAN Pack  CANdbFile=F:\PD\WHPC_PD\GateWay_20180620\CAN0_VehicleAllSignalWhAdd0530.dbc  MsgList=ESC2  MsgName=ESC2  MsgIDType=Standard (11-bit identifier)  MsgIdentifier=160  MsgLength=8  SignalInfo=ABS_ABSAlarm$27$1$2$2$1$0$1$0$-Inf$Inf$#ABS_EBDAlarm$24$1$2$2$1$0$1$0$-Inf$Inf$#ABS_VehSpd$56$16$2$2$1$0$1.000000e-002$0$-Inf$Inf$#ABS_VehSpdValidFlag$25$1$2$2$1$0$1$0$-Inf$Inf$#ABS_WorkLable$19$1$2$2$1$0$1$0$-Inf$Inf$#ESC_ABSValidity$26$1$2$2$1$0$1$0$0$1$#ESC_BrakeoilPress$13$11$2$1$1$0$1.000000e-002$0$0$17$#  NSignals=7  StartBits=str2num('[int32(27);int32(24);int32(56);int32(25);int32(19);int32(26);int32(13)]')  SignalSizes=str2num('[int32(1);int32(1);int32(16);int32(1);int32(1);int32(1);int32(11)]')  ByteOrders=str2num('[int32(2);int32(2);int32(2);int32(2);int32(2);int32(2);int32(2)]')  DataTypes=str2num('[int32(2);int32(2);int32(2);int32(2);int32(2);int32(2);int32(1)]')  MultiplexTypes=str2num('[int32(1);int32(1);int32(1);int32(1);int32(1);int32(1);int32(1)]')  MultiplexValues=str2num('[double(0);double(0);double(0);double(0);double(0);double(0);double(0)]')  Factors=str2num('[double(1);double(1);double(1.000000e-002);double(1);double(1);double(1);double(1.000000e-002)]')  Offsets=str2num('[double(0);double(0);double(0);double(0);double(0);double(0);double(0)]')  Minimums=str2num('[double(-Inf);double(-Inf);double(-Inf);double(-Inf);double(-Inf);double(0);double(0)]')  Maximums=str2num('[double(Inf);double(Inf);double(Inf);double(Inf);double(Inf);double(1);double(17)]')  Remote=off  ApplyMinMax=off  BusOutput=off
      settings: SourceProductName=Simulink Real-Time  SourceProductBaseCode=XP  DataFormat=CANdb specified signals
  CAN Send21 : S-Function  FunctionName=CAN_Send_P  Parameters=uint8(CAN_Port-1),uint8(CAN_Priority-1),uint8(S_overflow_flag),uint8(S_timestamp),double(sampletime)  SFunctionDeploymentMode=off  EnableBusSupport=off  mask{CAN_Port=CAN_0, CAN_Priority=3, S_overflow_flag=off, S_timestamp=off, sampletime=0.01}
      mask prompts: CAN_Port "CAN Port:"; CAN_Priority "Priority:"; S_overflow_flag "Send overflow flag"; S_timestamp "Send time stamp"
      mask init:
      | maskdisplay = cansendicon(CAN_Port,CAN_Priority,S_overflow_flag,S_timestamp);
      | set_param(gcb, 'MaskDisplay', maskdisplay);
      mask TypeOptions CAN_Port: CAN_0 | CAN_1 | CAN_2 | CAN_3
      mask TypeOptions CAN_Priority: 0 | 1 | 2 | 3 | 4 | 5 | 6 | 7
      mask Display: color('blue');text(0.98,0.9,'MPC5675K','horizontalAlignment','right');color('black');text(0.5,0.6,'FlexCAN_0 Send','horizontalAlignment','center');text(0.5,0.35,'Priority:3','horizontalAlignment','center');port_label('input',1,'CAN_Msg');
  Data Type Conversion75 : DataTypeConversion  OutDataTypeStr=single
  Data Type Conversion76 : DataTypeConversion  OutDataTypeStr=single
  Data Type Conversion{77..85} (9 alike) : DataTypeConversion  OutDataTypeStr=uint8
  Out1 : Outport
  Out2 : Outport  Port=2
  Out3 : Outport  Port=3
  Out4 : Outport  Port=4
  wires:
  Bus Selector13/7 -> Data Type Conversion81/1  "<LKA_action_indication>"
  Data Type Conversion78/1 -> CAN Pack21/4
  Bus Selector13/9 -> Data Type Conversion83/1  "<HMI_Popup_Status>"
  Bus Selector13/8 -> Data Type Conversion82/1  "<LKA_Status_Display>"
  Bus Selector13/10 -> Data Type Conversion84/1  "<Hands_off_warning>"
  Bus Selector13/4 -> Data Type Conversion78/1  "<Permit_to_know_if_LKA_or_LPA3F2>"
  Data Type Conversion83/1 -> Out2/1
  Data Type Conversion77/1 -> CAN Pack21/2
  Data Type Conversion84/1 -> Out3/1
  Data Type Conversion75/1 -> CAN Pack21/1
  Data Type Conversion79/1 -> CAN Pack21/5
  Data Type Conversion80/1 -> CAN Pack21/6
  Bus Selector13/11 -> Data Type Conversion85/1  "<Vehicle_Lane_Display>"
  Data Type Conversion81/1 -> CAN Pack21/7
  Bus Selector13/6 -> Data Type Conversion80/1  "<LDW_Status_Display>"
  Bus Selector13/3 -> Data Type Conversion76/1  "<Coefficient_toregulate_EPS>"
  CAN Pack21/1 -> CAN Send21/1
  Bus Selector13/2 -> Data Type Conversion77/1  "<EPS_State_Ctl>"
  Data Type Conversion76/1 -> CAN Pack21/3
  Bus Selector13/5 -> Data Type Conversion79/1  "<LDW_Flag>"
  [bsLLout] -> Bus Selector13/1
  Bus Selector13/1 -> Data Type Conversion75/1  "<LMS_phiSWACmd>"
  Data Type Conversion82/1 -> Out1/1
  Data Type Conversion85/1 -> Out4/1

== system D53_LKAS_JLU_20200909_1612/Clb/Calibration1 ==
  In1 : Inport
  In2 : Inport  Port=2
  Data Type Conversion{1..10} (10 alike) : DataTypeConversion  OutDataTypeStr=single
  If1 : If  IfExpression=u1 ==1  ElseIfExpressions=u1==2,u1==3,u1==4,u1==5,u1==6,u1==7,u1==8,u1==9,u1==10  ShowElse=off
  Rate Transition{1..3,5..11} (10 alike) : RateTransition  Deterministic=off  OutPortSampleTime=0.01
  Subsystem2 : Subsystem
  Out1 : Outport
  Out2 : Outport  Port=2
  Out3 : Outport  Port=3
  Out4 : Outport  Port=4
  Out5 : Outport  Port=5
  Out6 : Outport  Port=6
  Out7 : Outport  Port=7
  Out8 : Outport  Port=8
  Out9 : Outport  Port=9
  Out10 : Outport  Port=10
  wires:
  Subsystem2/10(Out10) -> Data Type Conversion10/1
  Subsystem2/4(Out4) -> Data Type Conversion4/1
  If1/3 -> Subsystem2/3(In3)
  Subsystem2/7(Out7) -> Data Type Conversion7/1
  Subsystem2/1(Out1) -> Data Type Conversion1/1
  Subsystem2/9(Out9) -> Data Type Conversion9/1
  If1/6 -> Subsystem2/6(In6)
  If1/2 -> Subsystem2/2(In2)
  If1/5 -> Subsystem2/5(In5)
  Subsystem2/8(Out8) -> Data Type Conversion8/1
  If1/9 -> Subsystem2/9(In9)
  If1/4 -> Subsystem2/4(In4)
  If1/1 -> Subsystem2/1(In1)
  If1/7 -> Subsystem2/7(In7)
  If1/8 -> Subsystem2/8(In8)
  Subsystem2/3(Out3) -> Data Type Conversion3/1
  Subsystem2/2(Out2) -> Data Type Conversion2/1
  If1/10 -> Subsystem2/10(In10)
  Subsystem2/5(Out5) -> Data Type Conversion5/1
  Subsystem2/6(Out6) -> Data Type Conversion6/1
  In1/1 -> If1/1
  In2/1 -> Subsystem2/11(In11)
  Data Type Conversion1/1 -> Rate Transition1/1
  Data Type Conversion2/1 -> Rate Transition2/1
  Data Type Conversion3/1 -> Rate Transition3/1
  Data Type Conversion4/1 -> Rate Transition5/1
  Data Type Conversion5/1 -> Rate Transition6/1
  Data Type Conversion6/1 -> Rate Transition7/1
  Data Type Conversion7/1 -> Rate Transition8/1
  Data Type Conversion8/1 -> Rate Transition9/1
  Data Type Conversion9/1 -> Rate Transition10/1
  Data Type Conversion10/1 -> Rate Transition11/1
  Rate Transition1/1 -> Out1/1
  Rate Transition2/1 -> Out2/1
  Rate Transition3/1 -> Out3/1
  Rate Transition5/1 -> Out4/1
  Rate Transition6/1 -> Out5/1
  Rate Transition7/1 -> Out6/1
  Rate Transition8/1 -> Out7/1
  Rate Transition9/1 -> Out8/1
  Rate Transition10/1 -> Out9/1
  Rate Transition11/1 -> Out10/1

== system D53_LKAS_JLU_20200909_1612/Clb/Calibration2 ==
  In1 : Inport
  In2 : Inport  Port=2
  Data Type Conversion{1..10} (10 alike) : DataTypeConversion  OutDataTypeStr=single
  If1 : If  IfExpression=u1 ==11  ElseIfExpressions=u1==12,u1==13,u1==14,u1==15,u1==16,u1==17,u1==18,u1==19,u1==20  ShowElse=off
  Rate Transition{1..3,5..11} (10 alike) : RateTransition  Deterministic=off  OutPortSampleTime=0.01
  Subsystem2 : Subsystem
  Out1 : Outport
  Out2 : Outport  Port=2
  Out3 : Outport  Port=3
  Out4 : Outport  Port=4
  Out5 : Outport  Port=5
  Out6 : Outport  Port=6
  Out7 : Outport  Port=7
  Out8 : Outport  Port=8
  Out9 : Outport  Port=9
  Out10 : Outport  Port=10
  wires:
  If1/10 -> Subsystem2/10(In10)
  If1/8 -> Subsystem2/8(In8)
  If1/7 -> Subsystem2/7(In7)
  If1/1 -> Subsystem2/1(In1)
  If1/4 -> Subsystem2/4(In4)
  If1/9 -> Subsystem2/9(In9)
  If1/5 -> Subsystem2/5(In5)
  If1/2 -> Subsystem2/2(In2)
  If1/6 -> Subsystem2/6(In6)
  If1/3 -> Subsystem2/3(In3)
  In2/1 -> Subsystem2/11(In11)
  In1/1 -> If1/1
  Data Type Conversion3/1 -> Rate Transition3/1
  Data Type Conversion2/1 -> Rate Transition2/1
  Data Type Conversion10/1 -> Rate Transition11/1
  Data Type Conversion5/1 -> Rate Transition6/1
  Rate Transition6/1 -> Out5/1
  Subsystem2/5(Out5) -> Data Type Conversion5/1
  Subsystem2/6(Out6) -> Data Type Conversion6/1
  Subsystem2/10(Out10) -> Data Type Conversion10/1
  Subsystem2/1(Out1) -> Data Type Conversion1/1
  Subsystem2/9(Out9) -> Data Type Conversion9/1
  Subsystem2/7(Out7) -> Data Type Conversion7/1
  Subsystem2/8(Out8) -> Data Type Conversion8/1
  Subsystem2/3(Out3) -> Data Type Conversion3/1
  Subsystem2/4(Out4) -> Data Type Conversion4/1
  Data Type Conversion4/1 -> Rate Transition5/1
  Data Type Conversion8/1 -> Rate Transition9/1
  Data Type Conversion9/1 -> Rate Transition10/1
  Data Type Conversion7/1 -> Rate Transition8/1
  Rate Transition8/1 -> Out7/1
  Rate Transition1/1 -> Out1/1
  Rate Transition2/1 -> Out2/1
  Rate Transition5/1 -> Out4/1
  Rate Transition10/1 -> Out9/1
  Rate Transition11/1 -> Out10/1
  Rate Transition3/1 -> Out3/1
  Subsystem2/2(Out2) -> Data Type Conversion2/1
  Data Type Conversion6/1 -> Rate Transition7/1
  Rate Transition7/1 -> Out6/1
  Data Type Conversion1/1 -> Rate Transition1/1
  Rate Transition9/1 -> Out8/1
